simulink model "skid_steer_controller"  (R2025a)
settings: Solver=ode4  StartTime=0.0  StopTime=10  FixedStep=0.01  RelTol=1e-3
libraries: simulink x1
settings Model: Creator=USER  LastModifiedBy=USER

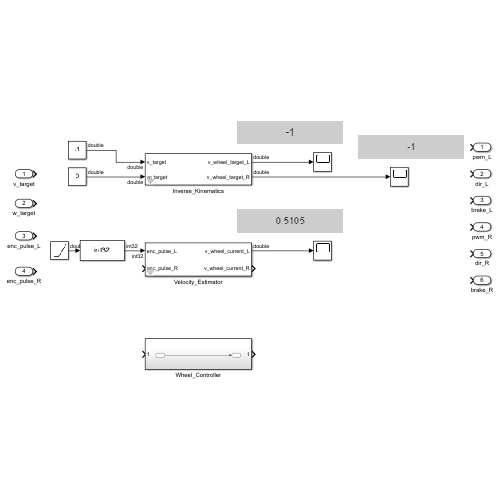
[thumbnail: Simulink's stored preview of the top-level diagram]
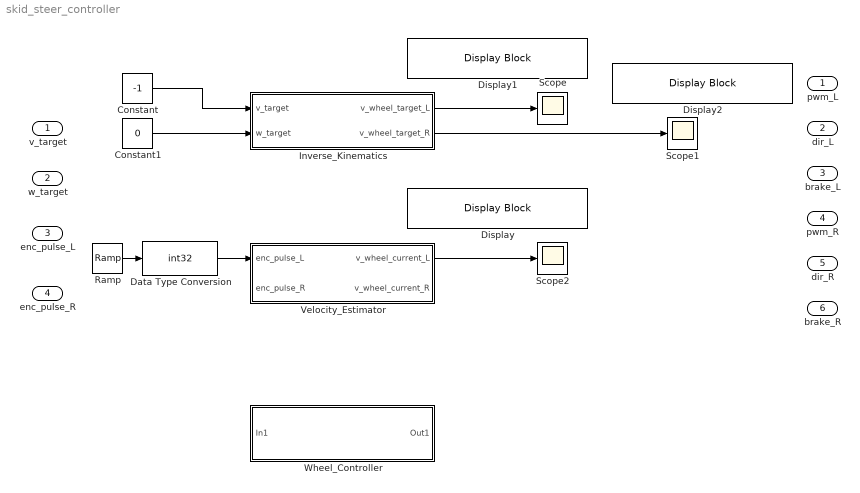
== system skid_steer_controller ==
  v_target : Inport
  w_target : Inport  Port=2
  enc_pulse_L : Inport  Port=3
  enc_pulse_R : Inport  Port=4
  Constant : Constant  Value=-1  OutDataTypeStr=double
  Constant1 : Constant  Value=0  OutDataTypeStr=double
  Data Type Conversion : DataTypeConversion  OutDataTypeStr=int32  SaturateOnIntegerOverflow=off  RndMeth=Floor
  Display : DisplayBlock  LabelPosition=Hide  Transparency=1  GridColor=[0.502, 0.502, 0.502]
  Display1 : DisplayBlock  LabelPosition=Hide  Transparency=1  GridColor=[0.502, 0.502, 0.502]
  Display2 : DisplayBlock  LabelPosition=Hide  Transparency=1  GridColor=[0.502, 0.502, 0.502]
  Inverse_Kinematics : Subsystem  mask{TRACK_WIDTH=0.25}
  Ramp : simulink/Sources/Ramp  slope=1000  start=0  InitialOutput=0
  Scope : Scope
      settings: ActiveDisplayYMinimum=-1.2831243491365227  ActiveDisplayYMaximum=2.7347801174971935
  Scope1 : Scope
      settings: ActiveDisplayYMinimum=-1.3008429866209543  ActiveDisplayYMaximum=2.0787462172836237
  Scope2 : Scope
      settings: ActiveDisplayYMinimum=-1  ActiveDisplayYMaximum=1  DataLoggingVariableName=ScopeData2
  Velocity_Estimator : Subsystem  mask{PPR=400, WHEEL_DIAMETER=0.065, SAMPLING_TIME=0.01}
      mask DialogControl ParameterGroupVar Prompt: 파라미터
  Wheel_Controller : Subsystem
  pwm_L : Outport
  dir_L : Outport  Port=2
  brake_L : Outport  Port=3
  pwm_R : Outport  Port=4
  dir_R : Outport  Port=5
  brake_R : Outport  Port=6
  wires:
  Inverse_Kinematics/1(v_wheel_target_L) -> Scope/1
  Inverse_Kinematics/2(v_wheel_target_R) -> Scope1/1
  Constant/1 -> Inverse_Kinematics/1(v_target)
  Constant1/1 -> Inverse_Kinematics/2(w_target)
  Ramp/1 -> Data Type Conversion/1
  Velocity_Estimator/1(v_wheel_current_L) -> Scope2/1
  Data Type Conversion/1 -> Velocity_Estimator/1(enc_pulse_L)

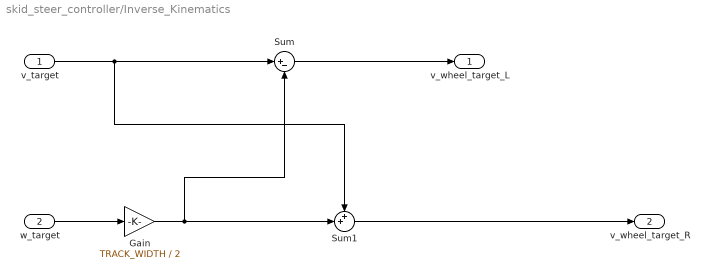
== system skid_steer_controller/Inverse_Kinematics ==
  v_target : Inport  OutDataTypeStr=double  Unit=m/s
  w_target : Inport  Port=2  OutDataTypeStr=double  Unit=rad/s
  Gain : Gain  Gain=TRACK_WIDTH / 2
  Sum : Sum  Inputs=|+-
  Sum1 : Sum  Inputs=++|
  v_wheel_target_L : Outport  OutDataTypeStr=double  Unit=m/s
  v_wheel_target_R : Outport  Port=2  OutDataTypeStr=double  Unit=m/s
  wires:
  Sum/1 -> v_wheel_target_L/1
  v_target/1 -> Sum1/1, Sum/1
  Sum1/1 -> v_wheel_target_R/1
  w_target/1 -> Gain/1
  Gain/1 -> Sum/2, Sum1/2

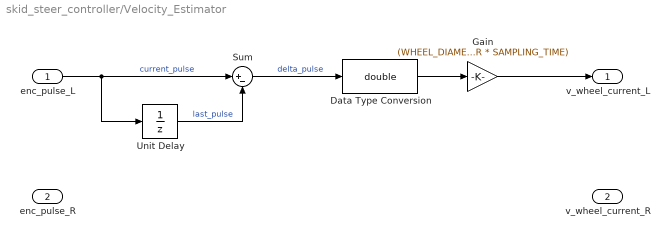
== system skid_steer_controller/Velocity_Estimator ==
  enc_pulse_L : Inport  OutDataTypeStr=int32  Unit=count
  enc_pulse_R : Inport  Port=2  OutDataTypeStr=int32  Unit=count
  Data Type Conversion : DataTypeConversion  OutDataTypeStr=double  SaturateOnIntegerOverflow=off  RndMeth=Floor
  Gain : Gain  Gain=(WHEEL_DIAMETER * pi) / (PPR * SAMPLING_TIME)
  Sum : Sum  Inputs=|+-
  Unit Delay : UnitDelay  SampleTime=-1  HasFrameUpgradeWarning=on
  v_wheel_current_L : Outport  OutDataTypeStr=double  Unit=m/s
  v_wheel_current_R : Outport  Port=2  OutDataTypeStr=double  Unit=m/s
  wires:
  enc_pulse_L/1 -> Sum/1, Unit Delay/1  "current_pulse"
  Unit Delay/1 -> Sum/2  "last_pulse"
  Sum/1 -> Data Type Conversion/1  "delta_pulse"
  Data Type Conversion/1 -> Gain/1
  Gain/1 -> v_wheel_current_L/1

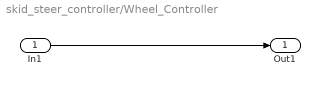
== system skid_steer_controller/Wheel_Controller ==
  In1 : Inport
  Out1 : Outport
  wires:
  In1/1 -> Out1/1
